simulink model "power_active_filter"  (R2017a)
settings: Solver=ode45  StartTime=0.0  StopTime=15/60  RelTol=1e-3  EnableMultiTasking=on
PreLoadFcn:
  | load power_active_filter.mat
InitFcn:
  | Ts=2e-6;
  | load power_active_filter.mat
undefined symbols (not defined in the file): AF, D1, Delta
libraries: powerlib x26
Description:
  | Copyright 2008-2017 The MathWorks, Inc.
settings Model: Creator=MathWorks  LastModifiedBy=Dell
settings DataIOCC: LimitDataPoints=on  SaveFormat=Array  SignalLoggingSaveFormat=ModelDataLogs
settings OptimizationCC: ExpressionDepthLimit=2147483647  InitFltsAndDblsToZero=on  LifeSpan=inf
settings DebuggingCC: SaveWithParameterizedLinksMsg=none  UnderspecifiedInitializationDetection=Classic  MergeDetectMultiDrivingBlocksExec=none  SignalResolutionControl=TryResolveAllWithWarning  SolverPrmCheckMsg=warning  MultiTaskDSMMsg=warning  MultiTaskCondExecSysMsg=none  FcnCallInpInsideContextMsg=warning  StateNameClashWarn=warning  SFUnexpectedBacktrackingDiag=warning  SFNoUnconditionalDefaultTransitionDiag=warning  SFExecutionAtInitializationDiag=none
settings HardwareCC: ProdBitPerPointer=32  ProdBitPerSizeT=32  ProdBitPerPtrDiffT=32  ProdLargestAtomicFloat=None  ProdIntDivRoundTo=Undefined  ProdEndianess=Unspecified  ProdWordSize=32  ProdHWDeviceType=32-bit Generic
settings ModelReferenceCC: PropagateSignalLabelsOutOfModel=off
settings GRTTargetCC: TargetFcnLib=ansi_tfl_tmw.mat  TargetLangStandard=C89/C90 (ANSI)  GeneratePreprocessorConditionals=Disable all  CombineOutputUpdateFcns=off  GRTInterface=on
settings ConfigComp: CovMetricSettings=dw  CovHtmlReporting=on  CovSaveCumulativeToWorkspaceVar=on  CovSaveSingleToWorkspaceVar=on  CovExternalEMLEnable=off  CovSFcnEnable=off

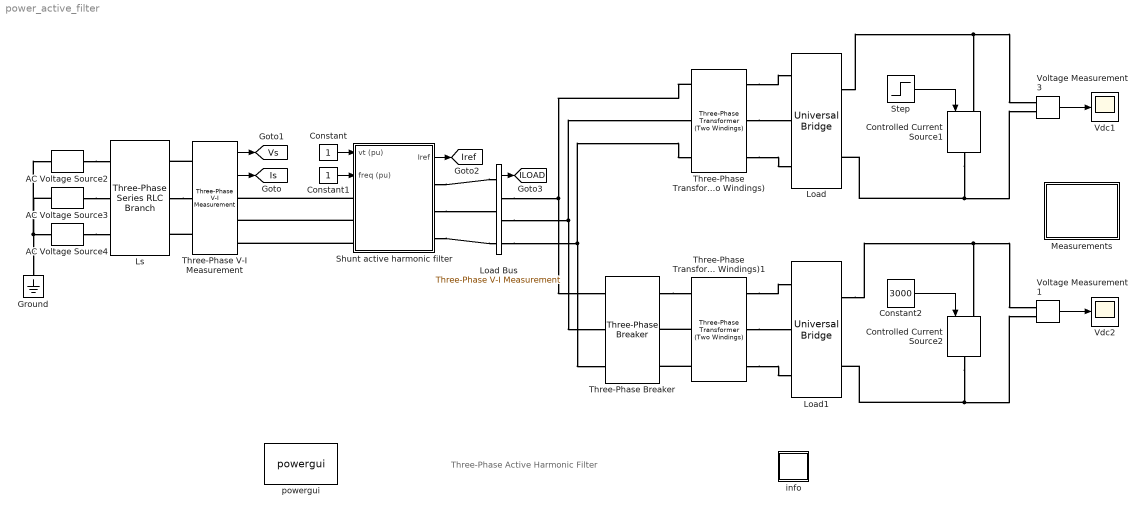
== system power_active_filter ==
  note: Three-Phase Active Harmonic Filter
  AC Voltage Source2 : powerlib/Electrical Sources/AC Voltage Source  Amplitude=4160*sqrt(2)/sqrt(3)  Phase=0  Frequency=60  SampleTime=0  Measurements=None  BusType=swing  Pref=10e3  Qref=0  Qmin=-inf  Qmax=+inf
  AC Voltage Source3 : powerlib/Electrical Sources/AC Voltage Source  Amplitude=4160*sqrt(2)/sqrt(3)  Phase=-120  Frequency=60  SampleTime=0  Measurements=None  BusType=swing  Pref=10e3  Qref=0  Qmin=-inf  Qmax=+inf
  AC Voltage Source4 : powerlib/Electrical Sources/AC Voltage Source  Amplitude=4160*sqrt(2)/sqrt(3)  Phase=120  Frequency=60  SampleTime=0  Measurements=None  BusType=swing  Pref=10e3  Qref=0  Qmin=-inf  Qmax=+inf
  Constant : Constant
  Constant1 : Constant
  Constant2 : Constant  Value=3000
  Controlled Current Source1 : powerlib/Electrical Sources/Controlled Current Source  Initialize=on  Source_Type=AC  Amplitude=0  Phase=0  Frequency=0  Measurements=None
  Controlled Current Source2 : powerlib/Electrical Sources/Controlled Current Source  Initialize=on  Source_Type=AC  Amplitude=0  Phase=0  Frequency=0  Measurements=None
  Ground : powerlib/Elements/Ground  LConnTagsString=a
  Load : powerlib/Power Electronics/Universal Bridge  Arms=3  SnubberResistance=1e3  SnubberCapacitance=1e-6  Device=Diodes  Ron=1e-3  Lon=0  ForwardVoltages="[  0  0  ]"  ForwardVoltage=0  GTOparameters=[ 10e-6 , 20e-6 ]  IGBTparameters=[ 1e-6 , 2e-6 ]  Measurements=None  Measurements_2=None  converterType=Rectifier
  Load Bus : powerlib/Measurements/Three-Phase V-I Measurement  VoltageMeasurement=no  SetLabelV=off  LabelV=Vabc  Vpu=off  VpuLL=off  CurrentMeasurement=yes  SetLabelI=off  LabelI=ILoad  Ipu=off  Pbase=100e6  Vbase=500e3  OutputType=Complex  PhasorSimulation=off  PSBequivalent=0
  Load1 : powerlib/Power Electronics/Universal Bridge  Arms=3  SnubberResistance=1e3  SnubberCapacitance=1e-6  Device=Diodes  Ron=1e-3  Lon=0  ForwardVoltages="[  0  0  ]"  ForwardVoltage=0  GTOparameters=[ 10e-6 , 20e-6 ]  IGBTparameters=[ 1e-6 , 2e-6 ]  Measurements=None  Measurements_2=None  converterType=Rectifier
  Ls : powerlib/Elements/Three-Phase Series RLC Branch  LConnTagsString=A|B|C  RConnTagsString=A|B|C  BranchType=L  Resistance=1  Inductance=1e-5  Capacitance=1e-6  Measurements=None
  Measurements : Subsystem
  Shunt active harmonic filter : Subsystem  mask(Parallel Active Filter){platform=AF}
  Step : Step  Time=5/60  Before=2000  After=3000  SampleTime=0
  Three-Phase Transformer (Two Windings) : powerlib/Elements/Three-Phase Transformer (Two Windings)  Winding1Connection=Delta (D1)  Winding2Connection=Delta (D1)  CoreType=Three single-phase transformers  SetSaturation=off  Hysteresis=off  DataFile='hysteresis'  SetInitialFlux=off  Measurements=None  UNITS=pu  NominalPower=[ 25e6 , 60 ]  Winding1=[4160, 0.002 , 0.08 ]  Winding2=[ 4160, 0.002 , 0.08 ]  Rm=500  Lm=500  L0=0.5  Saturation=[ 0,0 ; 0.0024,1.2 ; 1.0,1.52 ]  InitialFluxes=[ 0.8 , -0.8 , 0.7 ]  MoreParameters=off  BreakLoop=off  DataType=off  TransfoNumber=0
  Three-Phase Transformer (Two Windings)1 : powerlib/Elements/Three-Phase Transformer (Two Windings)  Winding1Connection=Delta (D1)  Winding2Connection=Y  CoreType=Three single-phase transformers  SetSaturation=off  Hysteresis=off  DataFile='hysteresis'  SetInitialFlux=off  Measurements=None  UNITS=pu  NominalPower=[ 25e6 , 60 ]  Winding1=[4160, 0.002 , 0.08 ]  Winding2=[ 4160, 0.002 , 0.08 ]  Rm=500  Lm=500  L0=0.5  Saturation=[ 0,0 ; 0.0024,1.2 ; 1.0,1.52 ]  InitialFluxes=[ 0.8 , -0.8 , 0.7 ]  MoreParameters=off  BreakLoop=off  DataType=off  TransfoNumber=0
  Three-Phase V-I Measurement : powerlib/Measurements/Three-Phase V-I Measurement  VoltageMeasurement=phase-to-ground  SetLabelV=off  LabelV=Vabc  Vpu=off  VpuLL=off  CurrentMeasurement=yes  SetLabelI=off  LabelI=Iabc  Ipu=off  Pbase=100e6  Vbase=500e3  OutputType=Complex  PhasorSimulation=off  PSBequivalent=0
  Three-Phase Breaker : powerlib/Elements/Three-Phase Breaker  InitialState=open  SwitchA=on  SwitchB=on  SwitchC=on  SwitchTimes=10/60  External=off  BreakerResistance=1e-5  SnubberResistance=1e6  SnubberCapacitance=inf  Measurements=None
  Vdc1 : Scope
  Vdc2 : Scope
  Voltage Measurement1 : powerlib/Measurements/Voltage Measurement  PhasorSimulation=off  OutputType=Complex  PSBequivalent=0
  Voltage Measurement3 : powerlib/Measurements/Voltage Measurement  PhasorSimulation=off  OutputType=Complex  PSBequivalent=0
  info : Subsystem
      settings: OpenFcn=showdemo(bdroot(gcb))
      mask Display: disp('?')
  powergui : powerlib/powergui  SimulationMode=Discrete  SampleTime=Ts  frequency=60  Iterations=50  frequencyindice=60  Pbase=100e6  ErrMax=1e-4  UnitsV=kV  UnitsW=MW  buscounter=0  FunctionMessages=off  echomessages=off  EnableUseOfTLC=off  CurrentSourceSwitches=off  DisableSnubberDevices=off  DisableRonSwitches=off  DisableVfSwitches=off  DisplayEquations=off  SolverType=Tustin/Backward Euler (TBE)  Interpol=off  ExternalGateDelay=off  methode=off  Ts=0  x0status=blocks  SPID=off  SwTol=0  HookPort=off  RestoreLinks=warning  ResistiveCurrentMeasurement=off  Frange=[0:2:500]  Ylog=off  Xlog=on  ShowGrid=off  save=off  variable=ZData  structure=Isource_Iload  ZoomFFT=on  StartTime=13/60  cycles=1  DisplayStyle=1  fundamental=60  FreqAxis=on  MaxFrequency=2000  frequencyindicesteady=1  RmsSteady=1  display=off
  tag scope: ILOAD=global, Iref=global, Is=global, Vs=global
  wires:
  Step/1 -> Controlled Current Source1/1
  Voltage Measurement3/1 -> Vdc1/1
  Constant/1 -> Shunt active harmonic filter/1(vt (pu))
  Constant1/1 -> Shunt active harmonic filter/2(freq (pu))
  Constant2/1 -> Controlled Current Source2/1
  Voltage Measurement1/1 -> Vdc2/1
  Three-Phase V-I Measurement/2 -> [Is]
  Three-Phase V-I Measurement/1 -> [Vs]
  Shunt active harmonic filter/1(Iref) -> [Iref]
  Load Bus/1 -> [ILOAD]
  connections:
  AC Voltage Source3/LConn1 -- AC Voltage Source2/LConn1 -- AC Voltage Source4/LConn1 -- Ground/LConn1
  AC Voltage Source2/RConn1 -- Ls/LConn1
  AC Voltage Source3/RConn1 -- Ls/LConn2
  AC Voltage Source4/RConn1 -- Ls/LConn3
  Three-Phase V-I Measurement/LConn1 -- Ls/RConn1
  Ls/RConn2 -- Three-Phase V-I Measurement/LConn2
  Three-Phase V-I Measurement/LConn3 -- Ls/RConn3
  Load/RConn1 -- Controlled Current Source1/LConn1 -- Voltage Measurement3/LConn1
  Controlled Current Source1/RConn1 -- Load/RConn2 -- Voltage Measurement3/LConn2
  Shunt active harmonic filter/LConn1 -- Three-Phase V-I Measurement/RConn1
  Shunt active harmonic filter/LConn2 -- Three-Phase V-I Measurement/RConn2
  Shunt active harmonic filter/LConn3 -- Three-Phase V-I Measurement/RConn3
  Three-Phase Breaker/RConn1 -- Three-Phase Transformer (Two Windings)1/LConn1
  Three-Phase Transformer (Two Windings)1/LConn2 -- Three-Phase Breaker/RConn2
  Three-Phase Transformer (Two Windings)1/LConn3 -- Three-Phase Breaker/RConn3
  Controlled Current Source2/RConn1 -- Voltage Measurement1/LConn2 -- Load1/RConn2
  Load1/RConn1 -- Voltage Measurement1/LConn1 -- Controlled Current Source2/LConn1
  Shunt active harmonic filter/RConn1 -- Load Bus/LConn1
  Shunt active harmonic filter/RConn2 -- Load Bus/LConn2
  Shunt active harmonic filter/RConn3 -- Load Bus/LConn3
  Three-Phase Transformer (Two Windings)/LConn1 -- Load Bus/RConn1 -- Three-Phase Breaker/LConn1
  Load Bus/RConn2 -- Three-Phase Transformer (Two Windings)/LConn2 -- Three-Phase Breaker/LConn2
  Load Bus/RConn3 -- Three-Phase Transformer (Two Windings)/LConn3 -- Three-Phase Breaker/LConn3
  Three-Phase Transformer (Two Windings)/RConn1 -- Load/LConn1
  Three-Phase Transformer (Two Windings)/RConn2 -- Load/LConn2
  Three-Phase Transformer (Two Windings)/RConn3 -- Load/LConn3
  Three-Phase Transformer (Two Windings)1/RConn1 -- Load1/LConn1
  Three-Phase Transformer (Two Windings)1/RConn2 -- Load1/LConn2
  Three-Phase Transformer (Two Windings)1/RConn3 -- Load1/LConn3

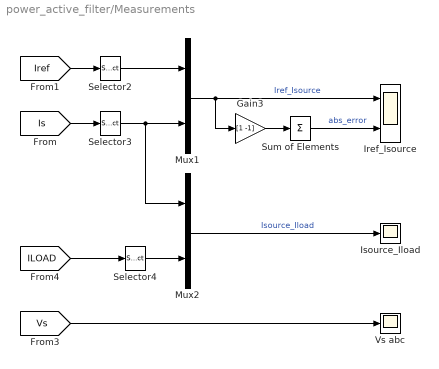
== system power_active_filter/Measurements ==
  Gain3 : Gain  Gain=[1 -1]
  Iref_Isource : Scope  NumInputPorts=2
  Isource_Iload : Scope
  Mux1 : Mux  Inputs=2
  Mux2 : Mux  Inputs=2
  Selector2 : Selector  InputPortWidth=3  IndexOptions=Index vector (dialog)  Indices=1  OutputSizes=1
  Selector3 : Selector  InputPortWidth=3  IndexOptions=Index vector (dialog)  Indices=1  OutputSizes=1
  Selector4 : Selector  InputPortWidth=3  IndexOptions=Index vector (dialog)  Indices=1  OutputSizes=1
  Sum of Elements : Sum  Inputs=+
  Vs abc : Scope
  wires:
  Mux1/1 -> Gain3/1, Iref_Isource/1  "Iref_Isource"
  Selector2/1 -> Mux1/1
  Selector3/1 -> Mux1/2, Mux2/1
  [Iref] -> Selector2/1
  [Is] -> Selector3/1
  Mux2/1 -> Isource_Iload/1  "Isource_Iload"
  Selector4/1 -> Mux2/2
  [ILOAD] -> Selector4/1
  Gain3/1 -> Sum of Elements/1
  Sum of Elements/1 -> Iref_Isource/2  "abs_error"
  [Vs] -> Vs abc/1

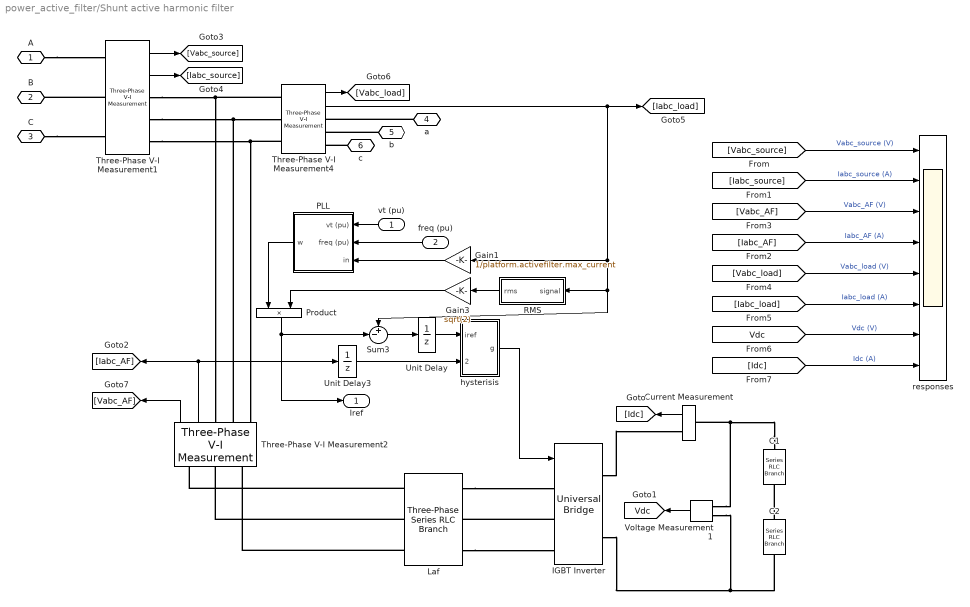
== system power_active_filter/Shunt active harmonic filter ==
  vt (pu) : Inport
  freq (pu) : Inport  Port=2
  C1 : powerlib/Elements/Series RLC Branch  LConnTagsString=__new0  RConnTagsString=__new0  BranchType=C  Resistance=1  Inductance=1e-3  SetiL0=off  InitialCurrent=0  Capacitance=platform.activefilter.DC_cap  Setx0=off  InitialVoltage=0  Measurements=None
  C2 : powerlib/Elements/Series RLC Branch  LConnTagsString=__new0  RConnTagsString=__new0  BranchType=C  Resistance=1  Inductance=1e-3  SetiL0=off  InitialCurrent=0  Capacitance=platform.activefilter.DC_cap  Setx0=off  InitialVoltage=0  Measurements=None
  Current Measurement : powerlib/Measurements/Current Measurement  PhasorSimulation=off  OutputType=Complex  PSBequivalent=0
  Gain1 : Gain  Gain=1/platform.activefilter.max_current
  Gain3 : Gain  Gain=sqrt(2)
  IGBT Inverter : powerlib/Power Electronics/Universal Bridge  Arms=3  SnubberResistance=platform.activefilter.bridge.Rs  SnubberCapacitance=platform.activefilter.bridge.Cs  Device=IGBT / Diodes  Ron=platform.activefilter.bridge.Ron  Lon=0  ForwardVoltages=platform.activefilter.bridge.Vf_Vfd  ForwardVoltage=0  GTOparameters=[ 10e-6 , 20e-6 ]  IGBTparameters=platform.activefilter.bridge.Tf_Ts  Measurements=None  Measurements_2=None  converterType=Rectifier
  Laf : powerlib/Elements/Three-Phase Series RLC Branch  LConnTagsString=A|B|C  RConnTagsString=A|B|C  BranchType=L  Resistance=1  Inductance=platform.activefilter.Laf  Capacitance=1e-6  Measurements=None
  PLL : Subsystem  mask{freq=platform.activefilter.freq}
      mask prompts: freq "Initial frequency (Hz)"
  Product : Product  RndMeth=Zero
  RMS : Subsystem  DialogController=POWERSYS.PowerSysDialog  mask(RMS){f1=platform.activefilter.freq}
      mask prompts: f1 "Fundamental frequency (Hz):"
      mask help: This block measures the root mean square value of instantaneous current or voltage signal connected to the input of the block. The RMS value is calculated over a running window of one cycle of the specified fundamental frequency.
      mask init:
      | power_initmask();
      mask Help: helpview(psbhelp)
  Sum3 : Sum  Inputs=+-|
  Three-Phase V-I Measurement1 : powerlib/Measurements/Three-Phase V-I Measurement  VoltageMeasurement=phase-to-phase  SetLabelV=off  LabelV=Vabc  Vpu=off  VpuLL=off  CurrentMeasurement=yes  SetLabelI=off  LabelI=Iabc  Ipu=off  Pbase=100e6  Vbase=500e3  OutputType=Complex  PhasorSimulation=off  PSBequivalent=0
  Three-Phase V-I Measurement2 : powerlib/Measurements/Three-Phase V-I Measurement  VoltageMeasurement=phase-to-phase  SetLabelV=off  LabelV=Vabc  Vpu=off  VpuLL=off  CurrentMeasurement=yes  SetLabelI=off  LabelI=Iabc  Ipu=off  Pbase=100e6  Vbase=500e3  OutputType=Complex  PhasorSimulation=off  PSBequivalent=0
  Three-Phase V-I Measurement4 : powerlib/Measurements/Three-Phase V-I Measurement  VoltageMeasurement=phase-to-phase  SetLabelV=off  LabelV=Vabc  Vpu=off  VpuLL=off  CurrentMeasurement=yes  SetLabelI=off  LabelI=Iabc  Ipu=off  Pbase=100e6  Vbase=500e3  OutputType=Complex  PhasorSimulation=off  PSBequivalent=0
  Unit Delay : UnitDelay  SampleTime=Ts
  Unit Delay3 : UnitDelay  SampleTime=Ts
  Voltage Measurement1 : powerlib/Measurements/Voltage Measurement  PhasorSimulation=off  OutputType=Complex  PSBequivalent=0
  hysterisis : Subsystem
  responses : Scope  NumInputPorts=8
  A : PMIOPort  Port=1  Side=Left
  B : PMIOPort  Port=2  Side=Left
  C : PMIOPort  Port=3  Side=Left
  a : PMIOPort  Port=4  Side=Right
  b : PMIOPort  Port=5  Side=Right
  c : PMIOPort  Port=6  Side=Right
  Iref : Outport
  tag scope: Vdc=global
  wires:
  Sum3/1 -> Unit Delay/1
  Three-Phase V-I Measurement2/2 -> Unit Delay3/1, [Iabc_AF]
  Unit Delay/1 -> hysterisis/1(iref)
  Unit Delay3/1 -> hysterisis/2(imeas)
  Current Measurement/1 -> [Idc]
  Three-Phase V-I Measurement4/2 -> Gain1/1, RMS/1(signal), Sum3/1, [Iabc_load]
  Product/1 -> Sum3/2, Iref/1
  RMS/1(rms) -> Gain3/1
  Voltage Measurement1/1 -> [Vdc]
  vt (pu)/1 -> PLL/1(vt (pu))
  Gain1/1 -> PLL/3(in)
  hysterisis/1(g) -> IGBT Inverter/1
  Three-Phase V-I Measurement2/1 -> [Vabc_AF]
  Three-Phase V-I Measurement4/1 -> [Vabc_load]
  Three-Phase V-I Measurement1/1 -> [Vabc_source]
  Three-Phase V-I Measurement1/2 -> [Iabc_source]
  PLL/1(w) -> Product/1
  Gain3/1 -> Product/2
  freq (pu)/1 -> PLL/2(freq (pu))
  [Vabc_source] -> responses/1  "Vabc_source (V)"
  [Iabc_source] -> responses/2  "Iabc_source (A)"
  [Vabc_AF] -> responses/3  "Vabc_AF (V)"
  [Iabc_AF] -> responses/4  "Iabc_AF (A)"
  [Vabc_load] -> responses/5  "Vabc_load (V)"
  [Iabc_load] -> responses/6  "Iabc_load (A)"
  [Vdc] -> responses/7  "Vdc (V)"
  [Idc] -> responses/8  "Idc (A)"
  connections:
  C1/LConn1 -- Voltage Measurement1/LConn1 -- Current Measurement/LConn1
  C2/LConn1 -- C1/RConn1
  C2/RConn1 -- Voltage Measurement1/LConn2 -- IGBT Inverter/RConn2
  IGBT Inverter/RConn1 -- Current Measurement/RConn1
  Laf/RConn1 -- IGBT Inverter/LConn1
  IGBT Inverter/LConn2 -- Laf/RConn2
  Laf/RConn3 -- IGBT Inverter/LConn3
  Laf/LConn1 -- Three-Phase V-I Measurement2/LConn1
  Laf/LConn2 -- Three-Phase V-I Measurement2/LConn2
  Laf/LConn3 -- Three-Phase V-I Measurement2/LConn3
  Three-Phase V-I Measurement4/LConn1 -- Three-Phase V-I Measurement2/RConn1 -- Three-Phase V-I Measurement1/RConn1
  Three-Phase V-I Measurement2/RConn2 -- Three-Phase V-I Measurement4/LConn2 -- Three-Phase V-I Measurement1/RConn2
  Three-Phase V-I Measurement4/LConn3 -- Three-Phase V-I Measurement2/RConn3 -- Three-Phase V-I Measurement1/RConn3
  a/RConn1 -- Three-Phase V-I Measurement4/RConn1
  b/RConn1 -- Three-Phase V-I Measurement4/RConn2
  c/RConn1 -- Three-Phase V-I Measurement4/RConn3
  C/RConn1 -- Three-Phase V-I Measurement1/LConn3
  Three-Phase V-I Measurement1/LConn2 -- B/RConn1
  A/RConn1 -- Three-Phase V-I Measurement1/LConn1

== system power_active_filter/info ==

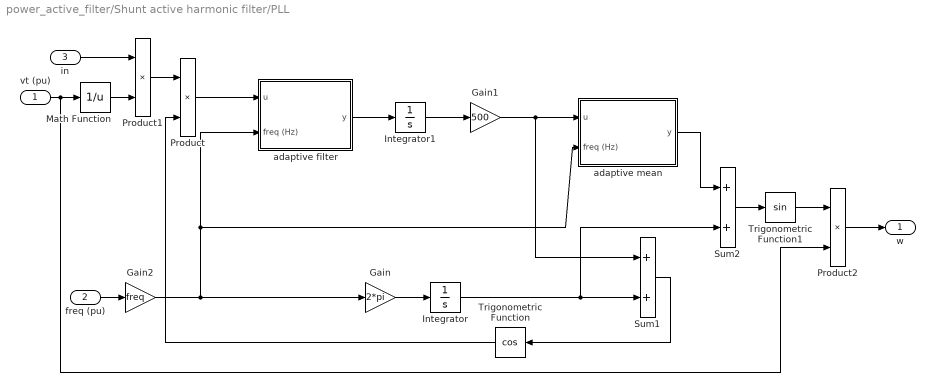
== system power_active_filter/Shunt active harmonic filter/PLL ==
  vt (pu) : Inport
  freq (pu) : Inport  Port=2
  in : Inport  Port=3
  Gain : Gain  Gain=2*pi
  Gain1 : Gain  Gain=500
  Gain2 : Gain  Gain=freq
  Integrator : Integrator
  Integrator1 : Integrator
  Math Function : Math  Operator=reciprocal  SaturateOnIntegerOverflow=on
  Product : Product  Inputs=**  RndMeth=Zero
  Product1 : Product  Inputs=**  RndMeth=Zero
  Product2 : Product  Inputs=**  RndMeth=Zero
  Sum1 : Sum  SaturateOnIntegerOverflow=on  InputSameDT=on  OutDataTypeStr=Inherit: Same as first input
  Sum2 : Sum  SaturateOnIntegerOverflow=on  InputSameDT=on  OutDataTypeStr=Inherit: Same as first input
  Trigonometric Function : Trigonometry  Operator=cos
  Trigonometric Function1 : Trigonometry
  adaptive filter : Subsystem
  adaptive mean : Subsystem
  w : Outport
  wires:
  freq (pu)/1 -> Gain2/1
  vt (pu)/1 -> Math Function/1, Product2/2
  Gain2/1 -> adaptive filter/2(freq (Hz)), adaptive mean/2(freq (Hz)), Gain/1
  Trigonometric Function/1 -> Product/2
  adaptive mean/1(y) -> Sum2/1
  Integrator1/1 -> Gain1/1
  Gain1/1 -> Sum1/1, adaptive mean/1(u)
  Integrator/1 -> Sum1/2, Sum2/2
  Gain/1 -> Integrator/1
  adaptive filter/1(y) -> Integrator1/1
  Product/1 -> adaptive filter/1(u)
  in/1 -> Product1/1
  Math Function/1 -> Product1/2
  Product1/1 -> Product/1
  Sum1/1 -> Trigonometric Function/1
  Sum2/1 -> Trigonometric Function1/1
  Trigonometric Function1/1 -> Product2/1
  Product2/1 -> w/1

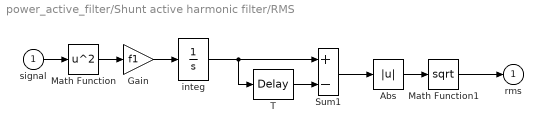
== system power_active_filter/Shunt active harmonic filter/RMS ==
  signal : Inport
  Abs : Abs  SaturateOnIntegerOverflow=on
  Gain : Gain  Gain=f1  SaturateOnIntegerOverflow=on  OutDataTypeStr=Inherit: Same as input  ParamDataTypeStr=Inherit: Same as input
  Math Function : Math  Operator=square  SaturateOnIntegerOverflow=on
  Math Function1 : Math  Operator=sqrt  SaturateOnIntegerOverflow=on
  Sum1 : Sum  Inputs=+-  SaturateOnIntegerOverflow=on  InputSameDT=on  OutDataTypeStr=Inherit: Same as first input
  T : TransportDelay  DelayTime=1/f1  BufferSize=9216
  integ : Integrator
  rms : Outport  InitialOutput=0
  wires:
  Gain/1 -> integ/1
  Math Function/1 -> Gain/1
  signal/1 -> Math Function/1
  Math Function1/1 -> rms/1
  integ/1 -> Sum1/1, T/1
  T/1 -> Sum1/2
  Sum1/1 -> Abs/1
  Abs/1 -> Math Function1/1

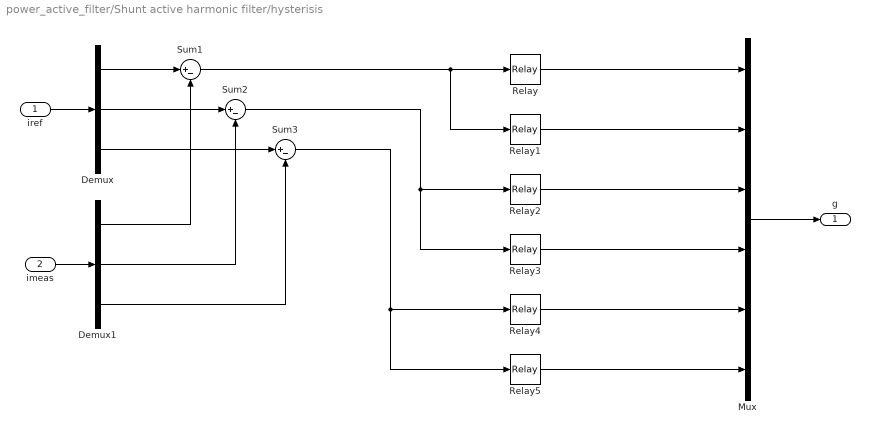
== system power_active_filter/Shunt active harmonic filter/hysterisis ==
  iref : Inport
  imeas : Inport  Port=2
  Demux : Demux  Outputs=3
  Demux1 : Demux  Outputs=3
  Mux : Mux  Inputs=6
  Relay : Relay
  Relay1 : Relay  OnOutputValue=0  OffOutputValue=1
  Relay2 : Relay
  Relay3 : Relay  OnOutputValue=0  OffOutputValue=1
  Relay4 : Relay
  Relay5 : Relay  OnOutputValue=0  OffOutputValue=1
  Sum1 : Sum  Inputs=|+-
  Sum2 : Sum  Inputs=|+-
  Sum3 : Sum  Inputs=|+-
  g : Outport
  wires:
  Mux/1 -> g/1
  iref/1 -> Demux/1
  imeas/1 -> Demux1/1
  Demux1/1 -> Sum1/2
  Demux1/2 -> Sum2/2
  Demux1/3 -> Sum3/2
  Demux/1 -> Sum1/1
  Demux/2 -> Sum2/1
  Demux/3 -> Sum3/1
  Sum1/1 -> Relay/1, Relay1/1
  Sum2/1 -> Relay2/1, Relay3/1
  Sum3/1 -> Relay5/1, Relay4/1
  Relay/1 -> Mux/1
  Relay1/1 -> Mux/2
  Relay2/1 -> Mux/3
  Relay3/1 -> Mux/4
  Relay4/1 -> Mux/5
  Relay5/1 -> Mux/6

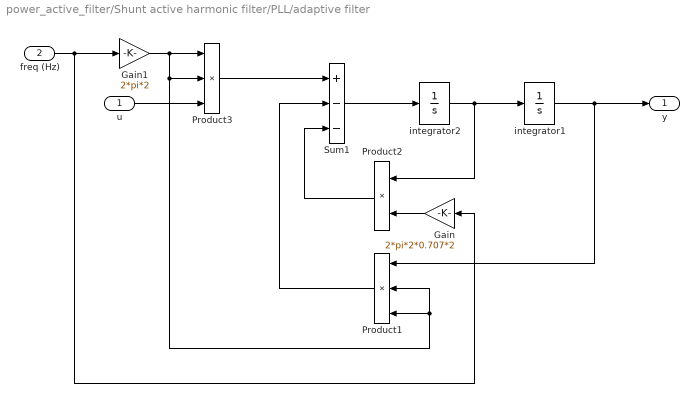
== system power_active_filter/Shunt active harmonic filter/PLL/adaptive filter ==
  u : Inport
  freq (Hz) : Inport  Port=2
  Gain : Gain  Gain=2*pi*2*0.707*2
  Gain1 : Gain  Gain=2*pi*2
  Product1 : Product  Inputs=***  RndMeth=Zero
  Product2 : Product  Inputs=**  RndMeth=Zero
  Product3 : Product  Inputs=***  RndMeth=Zero
  Sum1 : Sum  Inputs=+--  SaturateOnIntegerOverflow=on  InputSameDT=on  OutDataTypeStr=Inherit: Same as first input
  integrator1 : Integrator
  integrator2 : Integrator
  y : Outport
  wires:
  Product1/1 -> Sum1/2
  u/1 -> Product3/3
  freq (Hz)/1 -> Gain/1, Gain1/1
  Gain1/1 -> Product1/3, Product1/2, Product3/2, Product3/1
  Product3/1 -> Sum1/1
  integrator1/1 -> Product1/1, y/1
  Gain/1 -> Product2/2
  Product2/1 -> Sum1/3
  Sum1/1 -> integrator2/1
  integrator2/1 -> Product2/1, integrator1/1

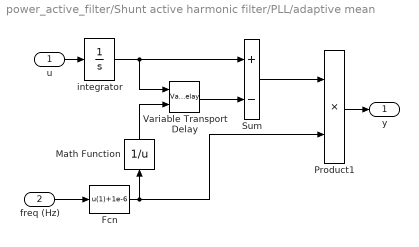
== system power_active_filter/Shunt active harmonic filter/PLL/adaptive mean ==
  u : Inport
  freq (Hz) : Inport  Port=2
  Fcn : Fcn  Expr=u(1)+1e-6
  Math Function : Math  Operator=reciprocal  SaturateOnIntegerOverflow=on
  Product1 : Product  Inputs=**  RndMeth=Zero
  Sum : Sum  Inputs=+-  SaturateOnIntegerOverflow=on  InputSameDT=on  OutDataTypeStr=Inherit: Same as first input
  Variable Transport Delay : VariableTransportDelay  MaximumDelay=1/40  MaximumPoints=16000
  integrator : Integrator
  y : Outport
  wires:
  Product1/1 -> y/1
  u/1 -> integrator/1
  Sum/1 -> Product1/1
  integrator/1 -> Variable Transport Delay/1, Sum/1
  Variable Transport Delay/1 -> Sum/2
  Math Function/1 -> Variable Transport Delay/2
  freq (Hz)/1 -> Fcn/1
  Fcn/1 -> Math Function/1, Product1/2
